simulink model "ModeAdjust"  (R2018b)
settings: Solver=FixedStepDiscrete  StartTime=0.0  StopTime=inf  FixedStep=0.01  RelTol=1e-3
undefined symbols (not defined in the file or in its folder): IfKeSMSbSeatMovBkRclnEnable_Val, IfKeSMSbSeatMovFrwdBkwdEnable_Val, IfKeSMSbSeatMovFtrstEnable_Val, IfKeSMSbSeatMovHdrstFrwdBkwdEnable_Val, IfKeSMSbSeatMovHdUpwdDnwdEnable_Val, IfKeSMSbSeatMovLgrstEnable_Val, IfKeSMSbSeatMovLtwdRtwdEnable_Val, IfVeSMSeStNumConfig, KeSMSbArmscreenMovEnable_Val, KeSMSbSeatMovLgrstExpdEnable_Val, KeSMSuFirstRwStBackPosDelta_Val, KeSMSuFirstRwStBackPosTolr_Val, KeSMSuFirstRwStCushFrntPosDelta_Val, KeSMSuFirstRwStCushFrntPosTolr_Val, KeSMSuFirstRwStCushRePosDelta_Val, KeSMSuFirstRwStCushRePosTolr_Val, KeSMSuFirstRwStFootrestPosDelta_Val, KeSMSuFirstRwStFootrestPosTolr_Val, KeSMSuFirstRwStFwdBkwdPosDelta_Val, KeSMSuFirstRwStFwdBkwdPosTolr_Val, KeSMSuMdMotFinshdTm_Val, KeSMSuMdRetryTm1_Val, KeSMSuModeReqDurgTm_Val, KeSMSuSecRwStArmTochPosDelta_Val, KeSMSuSecRwStArmTochPosTolr_Val, KeSMSuSecRwStBackPosDelta_Val, KeSMSuSecRwStBackPosTolr_Val, KeSMSuSecRwStFtrstUpwdDnwdPosDelta_Val, KeSMSuSecRwStFtrstUpwdDnwdPosTolr_Val, KeSMSuSecRwStFwdBkwdPosDelta_Val, KeSMSuSecRwStFwdBkwdPosTolr_Val, KeSMSuSecRwStHeadrestFwdBkwdPosDelta_Val, KeSMSuSecRwStHeadrestFwdBkwdPosTolr_Val, KeSMSuSecRwStHeadrestUpwdDwnwdPosDelta_Val, KeSMSuSecRwStHeadrestUpwdDwnwdPosTolr_Val, KeSMSuSecRwStLegrestInOutPosDelta_Val, KeSMSuSecRwStLegrestInOutPosTolr_Val, KeSMSuSecRwStLegrestUpwdDwnwdPosDelta_Val, KeSMSuSecRwStLegrestUpwdDwnwdPosTolr_Val, KeSMSuSecRwStLwdRwdPosDelta_Val, KeSMSuSecRwStLwdRwdPosTolr_Val, KeSMSuSecRwStVIPFtrstRefAngle_Val, KeSMSuThirdRwStFwdBkwdPosDelta_Val, KeSMSuThirdRwStFwdBkwdPosTolr_Val, KeSMSuThrdRwCushFoldPosDelta_Val, KeSMSuThrdRwCushFoldPosTolr_Val, KeSMSuThrdRwStBackPosDelta_Val, KeSMSuThrdRwStBackPosTolr_Val, KeSMSw4SLegrstCloseMdSecRwLtStFtrstUpwdDnwdPos_Val, KeSMSw4SLegrstCloseMdSecRwLtStFtrstUpwdDnwdPosMax_Val, KeSMSw4SLegrstCloseMdSecRwLtStFtrstUpwdDnwdPosMin_Val, KeSMSw4SLegrstCloseMdSecRwLtStLgrstOtwdInwdPos_Val, KeSMSw4SLegrstCloseMdSecRwLtStLgrstOtwdInwdPosMax_Val, KeSMSw4SLegrstCloseMdSecRwLtStLgrstOtwdInwdPosMin_Val, KeSMSw4SLegrstCloseMdSecRwLtStLgrstUpwdDnwdPos_Val, KeSMSw4SLegrstCloseMdSecRwLtStLgrstUpwdDnwdPosMax_Val, KeSMSw4SLegrstCloseMdSecRwLtStLgrstUpwdDnwdPosMin_Val, KeSMSw4SLegrstCloseMdSecRwRtStFtrstUpwdDnwdPos_Val, KeSMSw4SLegrstCloseMdSecRwRtStFtrstUpwdDnwdPosMax_Val, KeSMSw4SLegrstCloseMdSecRwRtStFtrstUpwdDnwdPosMin_Val ... (+1138)
libraries: Lib x401
(part 28 of 35)

== system ModeAdjust/ModeAdjustRunnable_sys/ModeAdjust/ArrivedAtTargetPosChk/Lug/R3Lt ==
  ThdRwLtStPoss : Inport
  ModeStCalib_3L : Inport  Port=2
  is6s : Inport  Port=3
  StConfig : Inport  Port=4
  IfVeSMSbThdRwLtStFrwdCmdSrv_Val_read : Inport  Port=5
  ThdRwLtStPossV : Inport  Port=6
  PosDeltaCalib : Inport  Port=7
  Bus Selector : BusSelector  OutputSignals=IfVeSMSuThdRwLtStBkReclnUpwdDnwdPos_Val_read,IfVeSMSuThdRwLtStCshnFldUpwdDnwdPos_Val_read,IfVeSMSuThdRwLtStFrwdBkwdPos_Val_read
  Bus Selector1 : BusSelector  OutputSignals=IfVeSMSuThdRwLtStBkReclnUpwdDnwdPosV_Val_read,IfVeSMSuThdRwLtStCshnFldUpwdDnwdPosV_Val_read,IfVeSMSuThdRwLtStFrwdBkwdPosV_Val_read
  Bus Selector2 : BusSelector  OutputSignals=BkReclnUpwdDnwdPos,BkReclnUpwdDnwdPosMax,BkReclnUpwdDnwdPosMin,CshnFldUpwdDnwdPos,CshnFldUpwdDnwdPosMax,CshnFldUpwdDnwdPosMin,FrwdBkwdPos,FrwdBkwdPosMax,FrwdBkwdPosMin
  Bus Selector3 : BusSelector  OutputSignals=LugThdRwLtSt
  Bus Selector4 : BusSelector  OutputSignals=BkReclnUpwdDnwdMovConfig,CshnFldUpwdDnwdMovConfig,FrwdBkwdMovConfig
  Bus Selector5 : BusSelector  OutputSignals=KeSMSuThirdRwStFwdBkwdPosDelta_Val,KeSMSuThrdRwCushFoldPosDelta_Val,KeSMSuThrdRwStBackPosDelta_Val
  CheckAtPos : Lib/CheckAtPos  SystemSampleTime=-1
  CheckAtPos1 : Lib/CheckAtPos  SystemSampleTime=-1
  CheckAtPos2 : Lib/CheckAtPos  SystemSampleTime=-1
  Constant{,1..4} (5 alike) : Constant  Value=0  OutDataTypeStr=boolean
  IsArrivedTarZone : Lib/CommonUsed/IniPosjudg/Subsystem2  SystemSampleTime=-1
  IsArrivedTarZone2 : Lib/CommonUsed/IniPosjudg/Subsystem2  SystemSampleTime=-1
  Logical Operator1 : Logic  Operator=NOT  AllPortsSameDT=off  OutDataTypeStr=boolean
  Logical Operator3 : Logic  Inputs=3  AllPortsSameDT=off  OutDataTypeStr=boolean
  R3Lt_ArrivedTarPos : Outport
  wires:
  Logical Operator3/1 -> R3Lt_ArrivedTarPos/1
  Bus Selector/1 -> [ThdRwLtStBkReclnUpwdDnwdPos]  "<IfVeSMSuThdRwLtStBkReclnUpwdDnwdPos_Val_read>"
  Bus Selector/3 -> [ThdRwLtStFrwdBkwdPos]  "<IfVeSMSuThdRwLtStFrwdBkwdPos_Val_read>"
  ThdRwLtStPoss/1 -> Bus Selector/1
  Bus Selector/2 -> [ThdRwLtStCshnFldUpwdDnwdPos]  "<IfVeSMSuThdRwLtStCshnFldUpwdDnwdPos_Val_read>"
  IsArrivedTarZone2/1 -> [Step3ArrivedTarPos]
  [ThdRwLtStCshnFldUpwdDnwdPos] -> IsArrivedTarZone2/1
  [K_CshnFldUpwdDnwdPosMin] -> IsArrivedTarZone2/2
  IsArrivedTarZone/1 -> [Step1ArrivedTarPos]
  [ThdRwLtStBkReclnUpwdDnwdPos] -> IsArrivedTarZone/1
  [K_BkReclnUpwdDnwdPosMin] -> IsArrivedTarZone/2
  [KeSMSuThrdRwStBackPosDelta_Val] -> IsArrivedTarZone/3
  [KeSMSuThrdRwCushFoldPosDelta_Val] -> IsArrivedTarZone2/3
  [K_BkReclnUpwdDnwdPosMax] -> IsArrivedTarZone/4
  [K_CshnFldUpwdDnwdPosMax] -> IsArrivedTarZone2/4
  Bus Selector2/6 -> [K_CshnFldUpwdDnwdPosMin]  "<CshnFldUpwdDnwdPosMin>"
  Bus Selector2/4 -> [K_CshnFldUpwdDnwdPos]  "<CshnFldUpwdDnwdPos>"
  Bus Selector2/7 -> [K_FrwdBkwdPos]  "<FrwdBkwdPos>"
  Bus Selector2/5 -> [K_CshnFldUpwdDnwdPosMax]  "<CshnFldUpwdDnwdPosMax>"
  ModeStCalib_3L/1 -> Bus Selector3/1
  Bus Selector2/3 -> [K_BkReclnUpwdDnwdPosMin]  "<BkReclnUpwdDnwdPosMin>"
  Bus Selector3/1 -> Bus Selector2/1  "<LugThdRwLtSt>"
  Bus Selector2/9 -> [K_FrwdBkwdPosMin]  "<FrwdBkwdPosMin>"
  Bus Selector2/2 -> [K_BkReclnUpwdDnwdPosMax]  "<BkReclnUpwdDnwdPosMax>"
  Bus Selector2/1 -> [K_BkReclnUpwdDnwdPos]  "<BkReclnUpwdDnwdPos>"
  Bus Selector2/8 -> [K_FrwdBkwdPosMax]  "<FrwdBkwdPosMax>"
  is6s/1 -> [is6s]
  Bus Selector4/1 -> [BkReclnUpwdDnwdMovConfig]  "<BkReclnUpwdDnwdMovConfig>"
  StConfig/1 -> Bus Selector4/1
  Bus Selector4/2 -> [CshnFldUpwdDnwdMovConfig]  "<CshnFldUpwdDnwdMovConfig>"
  Bus Selector4/3 -> [FrwdBkwdMovConfig]  "<FrwdBkwdMovConfig>"
  IfVeSMSbThdRwLtStFrwdCmdSrv_Val_read/1 -> Logical Operator1/1
  ThdRwLtStPossV/1 -> Bus Selector1/1
  Bus Selector1/3 -> [ThdRwLtStFrwdBkwdPosV]  "<IfVeSMSuThdRwLtStFrwdBkwdPosV_Val_read>"
  Bus Selector1/2 -> [ThdRwLtStCshnFldUpwdDnwdPosV]  "<IfVeSMSuThdRwLtStCshnFldUpwdDnwdPosV_Val_read>"
  Bus Selector1/1 -> [ThdRwLtStBkReclnUpwdDnwdPosV]  "<IfVeSMSuThdRwLtStBkReclnUpwdDnwdPosV_Val_read>"
  [BkReclnUpwdDnwdMovConfig] -> CheckAtPos/1
  [Step1ArrivedTarPos] -> CheckAtPos/3
  [FrwdBkwdMovConfig] -> CheckAtPos1/1
  Logical Operator1/1 -> CheckAtPos1/3
  [CshnFldUpwdDnwdMovConfig] -> CheckAtPos2/1
  [is6s] -> CheckAtPos2/5
  [Step3ArrivedTarPos] -> CheckAtPos2/3
  CheckAtPos1/1 -> Logical Operator3/2
  CheckAtPos2/1 -> Logical Operator3/3
  CheckAtPos/1 -> Logical Operator3/1
  [ThdRwLtStBkReclnUpwdDnwdPosV] -> CheckAtPos/2
  [ThdRwLtStCshnFldUpwdDnwdPosV] -> CheckAtPos2/2
  [ThdRwLtStFrwdBkwdPosV] -> CheckAtPos1/2
  Constant/1 -> CheckAtPos/4
  Constant1/1 -> CheckAtPos/5
  Constant2/1 -> CheckAtPos1/4
  Constant3/1 -> CheckAtPos1/5
  Constant4/1 -> CheckAtPos2/4
  Bus Selector5/1 -> [KeSMSuThirdRwStFwdBkwdPosDelta_Val]  "<KeSMSuThirdRwStFwdBkwdPosDelta_Val>"
  Bus Selector5/2 -> [KeSMSuThrdRwCushFoldPosDelta_Val]  "<KeSMSuThrdRwCushFoldPosDelta_Val>"
  Bus Selector5/3 -> [KeSMSuThrdRwStBackPosDelta_Val]  "<KeSMSuThrdRwStBackPosDelta_Val>"
  PosDeltaCalib/1 -> Bus Selector5/1

== system ModeAdjust/ModeAdjustRunnable_sys/ModeAdjust/ArrivedAtTargetPosChk/Lug/R3Rt ==
  ThdRwRtStPoss : Inport
  ModeStCalib_3R : Inport  Port=2
  is6s : Inport  Port=3
  StConfig : Inport  Port=4
  IfVeSMSbThdRwRtStFrwdCmdSrv_Val_read : Inport  Port=5
  ThdRwRtStPossV : Inport  Port=6
  PosDeltaCalib : Inport  Port=7
  Bus Selector : BusSelector  OutputSignals=IfVeSMSuThdRwRtStBkReclnUpwdDnwdPos_Val_read,IfVeSMSuThdRwRtStCshnFldUpwdDnwdPos_Val_read,IfVeSMSuThdRwRtStFrwdBkwdPos_Val_read
  Bus Selector1 : BusSelector  OutputSignals=IfVeSMSuThdRwRtStBkReclnUpwdDnwdPosV_Val_read,IfVeSMSuThdRwRtStCshnFldUpwdDnwdPosV_Val_read,IfVeSMSuThdRwRtStFrwdBkwdPosV_Val_read
  Bus Selector2 : BusSelector  OutputSignals=BkReclnUpwdDnwdPos,BkReclnUpwdDnwdPosMax,BkReclnUpwdDnwdPosMin,CshnFldUpwdDnwdPos,CshnFldUpwdDnwdPosMax,CshnFldUpwdDnwdPosMin,FrwdBkwdPos,FrwdBkwdPosMax,FrwdBkwdPosMin
  Bus Selector3 : BusSelector  OutputSignals=LugThdRwRtSt
  Bus Selector4 : BusSelector  OutputSignals=BkReclnUpwdDnwdMovConfig,CshnFldUpwdDnwdMovConfig,FrwdBkwdMovConfig
  Bus Selector5 : BusSelector  OutputSignals=KeSMSuThirdRwStFwdBkwdPosDelta_Val,KeSMSuThrdRwCushFoldPosDelta_Val,KeSMSuThrdRwStBackPosDelta_Val
  CheckAtPos : Lib/CheckAtPos  SystemSampleTime=-1
  CheckAtPos1 : Lib/CheckAtPos  SystemSampleTime=-1
  CheckAtPos2 : Lib/CheckAtPos  SystemSampleTime=-1
  Constant{,1..4} (5 alike) : Constant  Value=0  OutDataTypeStr=boolean
  IsArrivedTarZone : Lib/CommonUsed/IniPosjudg/Subsystem2  SystemSampleTime=-1
  IsArrivedTarZone2 : Lib/CommonUsed/IniPosjudg/Subsystem2  SystemSampleTime=-1
  Logical Operator1 : Logic  Operator=NOT  AllPortsSameDT=off  OutDataTypeStr=boolean
  Logical Operator3 : Logic  Inputs=3  AllPortsSameDT=off  OutDataTypeStr=boolean
  R3Rt_ArrivedTarPos : Outport
  wires:
  Logical Operator3/1 -> R3Rt_ArrivedTarPos/1
  Bus Selector/1 -> [ThdRwRtStBkReclnUpwdDnwdPos]  "<IfVeSMSuThdRwRtStBkReclnUpwdDnwdPos_Val_read>"
  Bus Selector/2 -> [ThdRwRtStCshnFldUpwdDnwdPos]  "<IfVeSMSuThdRwRtStCshnFldUpwdDnwdPos_Val_read>"
  ThdRwRtStPoss/1 -> Bus Selector/1
  Bus Selector/3 -> [ThdRwRtStFrwdBkwdPos]  "<IfVeSMSuThdRwRtStFrwdBkwdPos_Val_read>"
  [ThdRwRtStBkReclnUpwdDnwdPos] -> IsArrivedTarZone/1
  IsArrivedTarZone/1 -> [Step1ArrivedTarPos]
  [K_CshnFldUpwdDnwdPosMin] -> IsArrivedTarZone2/2
  [ThdRwRtStCshnFldUpwdDnwdPos] -> IsArrivedTarZone2/1
  IsArrivedTarZone2/1 -> [Step3ArrivedTarPos]
  [K_BkReclnUpwdDnwdPosMin] -> IsArrivedTarZone/2
  [KeSMSuThrdRwStBackPosDelta_Val] -> IsArrivedTarZone/3
  [KeSMSuThrdRwCushFoldPosDelta_Val] -> IsArrivedTarZone2/3
  [K_BkReclnUpwdDnwdPosMax] -> IsArrivedTarZone/4
  [K_CshnFldUpwdDnwdPosMax] -> IsArrivedTarZone2/4
  Bus Selector2/6 -> [K_CshnFldUpwdDnwdPosMin]  "<CshnFldUpwdDnwdPosMin>"
  Bus Selector2/4 -> [K_CshnFldUpwdDnwdPos]  "<CshnFldUpwdDnwdPos>"
  Bus Selector2/7 -> [K_FrwdBkwdPos]  "<FrwdBkwdPos>"
  Bus Selector2/5 -> [K_CshnFldUpwdDnwdPosMax]  "<CshnFldUpwdDnwdPosMax>"
  ModeStCalib_3R/1 -> Bus Selector3/1
  Bus Selector2/3 -> [K_BkReclnUpwdDnwdPosMin]  "<BkReclnUpwdDnwdPosMin>"
  Bus Selector3/1 -> Bus Selector2/1  "<LugThdRwRtSt>"
  Bus Selector2/9 -> [K_FrwdBkwdPosMin]  "<FrwdBkwdPosMin>"
  Bus Selector2/2 -> [K_BkReclnUpwdDnwdPosMax]  "<BkReclnUpwdDnwdPosMax>"
  Bus Selector2/1 -> [K_BkReclnUpwdDnwdPos]  "<BkReclnUpwdDnwdPos>"
  Bus Selector2/8 -> [K_FrwdBkwdPosMax]  "<FrwdBkwdPosMax>"
  is6s/1 -> [is6s]
  Bus Selector4/1 -> [BkReclnUpwdDnwdMovConfig]  "<BkReclnUpwdDnwdMovConfig>"
  StConfig/1 -> Bus Selector4/1
  Bus Selector4/2 -> [CshnFldUpwdDnwdMovConfig]  "<CshnFldUpwdDnwdMovConfig>"
  Bus Selector4/3 -> [FrwdBkwdMovConfig]  "<FrwdBkwdMovConfig>"
  IfVeSMSbThdRwRtStFrwdCmdSrv_Val_read/1 -> Logical Operator1/1
  ThdRwRtStPossV/1 -> Bus Selector1/1
  Bus Selector1/1 -> [ThdRwRtStBkReclnUpwdDnwdPosV]  "<IfVeSMSuThdRwRtStBkReclnUpwdDnwdPosV_Val_read>"
  Bus Selector1/3 -> [ThdRwRtStFrwdBkwdPosV]  "<IfVeSMSuThdRwRtStFrwdBkwdPosV_Val_read>"
  Bus Selector1/2 -> [ThdRwRtStCshnFldUpwdDnwdPosV]  "<IfVeSMSuThdRwRtStCshnFldUpwdDnwdPosV_Val_read>"
  CheckAtPos1/1 -> Logical Operator3/2
  CheckAtPos2/1 -> Logical Operator3/3
  CheckAtPos/1 -> Logical Operator3/1
  [BkReclnUpwdDnwdMovConfig] -> CheckAtPos/1
  [Step1ArrivedTarPos] -> CheckAtPos/3
  Logical Operator1/1 -> CheckAtPos1/3
  [FrwdBkwdMovConfig] -> CheckAtPos1/1
  [CshnFldUpwdDnwdMovConfig] -> CheckAtPos2/1
  [is6s] -> CheckAtPos2/5
  [Step3ArrivedTarPos] -> CheckAtPos2/3
  [ThdRwRtStBkReclnUpwdDnwdPosV] -> CheckAtPos/2
  [ThdRwRtStCshnFldUpwdDnwdPosV] -> CheckAtPos2/2
  [ThdRwRtStFrwdBkwdPosV] -> CheckAtPos1/2
  Constant/1 -> CheckAtPos/4
  Constant1/1 -> CheckAtPos/5
  Constant2/1 -> CheckAtPos1/4
  Constant3/1 -> CheckAtPos1/5
  Constant4/1 -> CheckAtPos2/4
  Bus Selector5/1 -> [KeSMSuThirdRwStFwdBkwdPosDelta_Val]  "<KeSMSuThirdRwStFwdBkwdPosDelta_Val>"
  Bus Selector5/2 -> [KeSMSuThrdRwCushFoldPosDelta_Val]  "<KeSMSuThrdRwCushFoldPosDelta_Val>"
  Bus Selector5/3 -> [KeSMSuThrdRwStBackPosDelta_Val]  "<KeSMSuThrdRwStBackPosDelta_Val>"
  PosDeltaCalib/1 -> Bus Selector5/1

== system ModeAdjust/ModeAdjustRunnable_sys/ModeAdjust/ArrivedAtTargetPosChk/Lug/Subsystem1 ==
  Left_inport : Inport
  Right_inport : Inport  Port=2
  Md_L_MvDoneOK : Outport
  Md_R_MvDoneOK : Outport  Port=2
  wires:
  Left_inport/1 -> Md_L_MvDoneOK/1
  Right_inport/1 -> Md_R_MvDoneOK/1

== system ModeAdjust/ModeAdjustRunnable_sys/ModeAdjust/ArrivedAtTargetPosChk/Ly/R2Lt ==
  SecRwLtStsPoss : Inport
  ModeStCalib_2L : Inport  Port=2
  StConfig : Inport  Port=3
  SecRwLtStsPoss4s : Inport  Port=4
  StConfig4s : Inport  Port=5
  SecRwLtStPossV : Inport  Port=6
  SecRwLtStPossV4s : Inport  Port=7
  Lt4sHightIndex : Inport  Port=8
  PosDeltaCalib : Inport  Port=9
  Bus Creator{,1..6} (7 alike) : BusCreator  Inputs=9
  Bus Selector : BusSelector  OutputSignals=IfVeSMSuSecRwLtStBkReclnUpwdDnwdPos_Val_read,IfVeSMSuSecRwLtStFrwdBkwdPos_Val_read,IfVeSMSuSecRwLtStHPassStUpwdDnwdPos_Val_read,IfVeSMSuSecRwLtStLgrstUpwdDnwdPos_Val_read,IfVeSMSuSecRwLtStLtwdRtwdPos_Val_read,IfVeSMSuSecRwLtStArmScrnPos_Val_read
  Bus Selector1 : BusSelector  OutputSignals=IfVeSMSuSecRwLtStLgrstOtwdInwdPos_Val_read,IfVeSMSuRrLtStFtUpwdDnwdPos_Val_read,IfVeSMSuSecRwLtStHdrstFrwdBkwdPos_Val_read
  Bus Selector2 : BusSelector  OutputSignals=BkReclnUpwdDnwdPosMax,BkReclnUpwdDnwdPosMin,LgrstUpwdPosMax,LgrstUpwdPosMin,FtrstUpwdDnwdPosMax,FtrstUpwdDnwdPosMin
  Bus Selector3 : BusSelector  OutputSignals=LyLSecRwLtSt
  Bus Selector4 : BusSelector  OutputSignals=BkReclnUpwdDnwdMovConfig,ArmTouchMovConfig,FrwdBkwdMovConfig,LgrstUpwdMovConfig,LtwdRtwdMovConfig
  Bus Selector5 : BusSelector  OutputSignals=LgrstExpdMovConfig,FtrstMovConfig,HdrstUpwdDnwdMovConfig,HdrstFrwdBkwdMovConfig
  Bus Selector6 : BusSelector  OutputSignals=IfVeSMSuSecRwLtStBkReclnUpwdDnwdPosV_Val_read,IfVeSMSuSecRwLtStFrwdBkwdPosV_Val_read,IfVeSMSuSecRwLtStHPassStUpwdDnwdPosV_Val_read,IfVeSMSuSecRwLtStLgrstUpwdDnwdPosV_Val_read,IfVeSMSuSecRwLtStLtwdRtwdPosV_Val_read,IfVeSMSuSecRwLtStArmScrnPosV_Val_read
  Bus Selector7 : BusSelector  OutputSignals=IfVeSMSuSecRwLtStLgrstOtwdInwdPosV_Val_read,IfVeSMSuRrLtStFtUpwdDnwdPosV_Val_read,IfVeSMSuSecRwLtStHdrstFrwdBkwdPosV_Val_read
  Bus Selector8 : BusSelector  OutputSignals=HdrstUpwdDnwdPosMax,HdrstUpwdDnwdPosMin,HdrstFrwdBkwdnwdPosMax,HdrstFrwdBkwdnwdPosMin,LgrstOtwdInwdPosMax,LgrstOtwdInwdPosMin
  Bus Selector9 : BusSelector  OutputSignals=KeSMSuSecRwStHeadrestFwdBkwdPosDelta_Val,KeSMSuSecRwStHeadrestUpwdDwnwdPosDelta_Val,KeSMSuSecRwStLegrestInOutPosDelta_Val,KeSMSuSecRwStFtrstUpwdDnwdPosDelta_Val,KeSMSuSecRwStBackPosDelta_Val,KeSMSuSecRwStLegrestUpwdDwnwdPosDelta_Val
  CheckAtPos{,1..5} (6 alike) : Lib/CheckAtPos  SystemSampleTime=-1
  Constant{1..12} (12 alike) : Constant  Value=0  OutDataTypeStr=boolean
  IsArrivedTarZone{,1..5} (6 alike) : Lib/CommonUsed/IniPosjudg/Subsystem2  SystemSampleTime=-1
  Logical Operator9 : Logic  Inputs=6  AllPortsSameDT=off  OutDataTypeStr=boolean
  Multiport Switch : MultiPortSwitch  DataPortOrder=Zero-based contiguous  Inputs=7  DiagnosticForDefault=None  zeroidx=on
  PA_KeSMSw4sLyingMDSecRwLtStHdrstFrwdBkwdnwdPosMax_160_Val : Constant  Value=KeSMSw4sLyingMDSecRwLtStHdrstFrwdBkwdnwdPosMax_160_Val
  PA_KeSMSw4sLyingMDSecRwLtStHdrstFrwdBkwdnwdPosMax_165_Val : Constant  Value=KeSMSw4sLyingMDSecRwLtStHdrstFrwdBkwdnwdPosMax_165_Val
  PA_KeSMSw4sLyingMDSecRwLtStHdrstFrwdBkwdnwdPosMax_170_Val : Constant  Value=KeSMSw4sLyingMDSecRwLtStHdrstFrwdBkwdnwdPosMax_170_Val
  PA_KeSMSw4sLyingMDSecRwLtStHdrstFrwdBkwdnwdPosMax_175_Val : Constant  Value=KeSMSw4sLyingMDSecRwLtStHdrstFrwdBkwdnwdPosMax_175_Val
  PA_KeSMSw4sLyingMDSecRwLtStHdrstFrwdBkwdnwdPosMax_180_Val : Constant  Value=KeSMSw4sLyingMDSecRwLtStHdrstFrwdBkwdnwdPosMax_180_Val
  PA_KeSMSw4sLyingMDSecRwLtStHdrstFrwdBkwdnwdPosMax_Below160_Val : Constant  Value=KeSMSw4sLyingMDSecRwLtStHdrstFrwdBkwdnwdPosMax_Below160_Val
  PA_KeSMSw4sLyingMDSecRwLtStHdrstFrwdBkwdnwdPosMax_Over180_Val : Constant  Value=KeSMSw4sLyingMDSecRwLtStHdrstFrwdBkwdnwdPosMax_Over180_Val
  PA_KeSMSw4sLyingMDSecRwLtStHdrstFrwdBkwdnwdPosMin_160_Val : Constant  Value=KeSMSw4sLyingMDSecRwLtStHdrstFrwdBkwdnwdPosMin_160_Val
  PA_KeSMSw4sLyingMDSecRwLtStHdrstFrwdBkwdnwdPosMin_165_Val : Constant  Value=KeSMSw4sLyingMDSecRwLtStHdrstFrwdBkwdnwdPosMin_165_Val
  PA_KeSMSw4sLyingMDSecRwLtStHdrstFrwdBkwdnwdPosMin_170_Val : Constant  Value=KeSMSw4sLyingMDSecRwLtStHdrstFrwdBkwdnwdPosMin_170_Val
  PA_KeSMSw4sLyingMDSecRwLtStHdrstFrwdBkwdnwdPosMin_175_Val : Constant  Value=KeSMSw4sLyingMDSecRwLtStHdrstFrwdBkwdnwdPosMin_175_Val
  PA_KeSMSw4sLyingMDSecRwLtStHdrstFrwdBkwdnwdPosMin_180_Val : Constant  Value=KeSMSw4sLyingMDSecRwLtStHdrstFrwdBkwdnwdPosMin_180_Val
  PA_KeSMSw4sLyingMDSecRwLtStHdrstFrwdBkwdnwdPosMin_Below160_Val : Constant  Value=KeSMSw4sLyingMDSecRwLtStHdrstFrwdBkwdnwdPosMin_Below160_Val
  PA_KeSMSw4sLyingMDSecRwLtStHdrstFrwdBkwdnwdPosMin_Over180_Val : Constant  Value=KeSMSw4sLyingMDSecRwLtStHdrstFrwdBkwdnwdPosMin_Over180_Val
  PA_KeSMSw4sLyingMDSecRwLtStHdrstFrwdBkwdnwdPos_160_Val : Constant  Value=KeSMSw4sLyingMDSecRwLtStHdrstFrwdBkwdnwdPos_160_Val
  PA_KeSMSw4sLyingMDSecRwLtStHdrstFrwdBkwdnwdPos_165_Val : Constant  Value=KeSMSw4sLyingMDSecRwLtStHdrstFrwdBkwdnwdPos_165_Val
  PA_KeSMSw4sLyingMDSecRwLtStHdrstFrwdBkwdnwdPos_170_Val : Constant  Value=KeSMSw4sLyingMDSecRwLtStHdrstFrwdBkwdnwdPos_170_Val
  PA_KeSMSw4sLyingMDSecRwLtStHdrstFrwdBkwdnwdPos_175_Val : Constant  Value=KeSMSw4sLyingMDSecRwLtStHdrstFrwdBkwdnwdPos_175_Val
  PA_KeSMSw4sLyingMDSecRwLtStHdrstFrwdBkwdnwdPos_180_Val : Constant  Value=KeSMSw4sLyingMDSecRwLtStHdrstFrwdBkwdnwdPos_180_Val
  PA_KeSMSw4sLyingMDSecRwLtStHdrstFrwdBkwdnwdPos_Below160_Val : Constant  Value=KeSMSw4sLyingMDSecRwLtStHdrstFrwdBkwdnwdPos_Below160_Val
  PA_KeSMSw4sLyingMDSecRwLtStHdrstFrwdBkwdnwdPos_Over180_Val : Constant  Value=KeSMSw4sLyingMDSecRwLtStHdrstFrwdBkwdnwdPos_Over180_Val
  PA_KeSMSw4sLyingMDSecRwLtStHdrstUpwdDnwdPosMax_160_Val : Constant  Value=KeSMSw4sLyingMDSecRwLtStHdrstUpwdDnwdPosMax_160_Val
  PA_KeSMSw4sLyingMDSecRwLtStHdrstUpwdDnwdPosMax_165_Val : Constant  Value=KeSMSw4sLyingMDSecRwLtStHdrstUpwdDnwdPosMax_165_Val
  PA_KeSMSw4sLyingMDSecRwLtStHdrstUpwdDnwdPosMax_170_Val : Constant  Value=KeSMSw4sLyingMDSecRwLtStHdrstUpwdDnwdPosMax_170_Val
  PA_KeSMSw4sLyingMDSecRwLtStHdrstUpwdDnwdPosMax_175_Val : Constant  Value=KeSMSw4sLyingMDSecRwLtStHdrstUpwdDnwdPosMax_175_Val
  PA_KeSMSw4sLyingMDSecRwLtStHdrstUpwdDnwdPosMax_180_Val : Constant  Value=KeSMSw4sLyingMDSecRwLtStHdrstUpwdDnwdPosMax_180_Val
  PA_KeSMSw4sLyingMDSecRwLtStHdrstUpwdDnwdPosMax_Below160_Val : Constant  Value=KeSMSw4sLyingMDSecRwLtStHdrstUpwdDnwdPosMax_Below160_Val
  PA_KeSMSw4sLyingMDSecRwLtStHdrstUpwdDnwdPosMax_Over180_Val : Constant  Value=KeSMSw4sLyingMDSecRwLtStHdrstUpwdDnwdPosMax_Over180_Val
  PA_KeSMSw4sLyingMDSecRwLtStHdrstUpwdDnwdPosMin_160_Val : Constant  Value=KeSMSw4sLyingMDSecRwLtStHdrstUpwdDnwdPosMin_160_Val
  PA_KeSMSw4sLyingMDSecRwLtStHdrstUpwdDnwdPosMin_165_Val : Constant  Value=KeSMSw4sLyingMDSecRwLtStHdrstUpwdDnwdPosMin_165_Val
  PA_KeSMSw4sLyingMDSecRwLtStHdrstUpwdDnwdPosMin_170_Val : Constant  Value=KeSMSw4sLyingMDSecRwLtStHdrstUpwdDnwdPosMin_170_Val
  PA_KeSMSw4sLyingMDSecRwLtStHdrstUpwdDnwdPosMin_175_Val : Constant  Value=KeSMSw4sLyingMDSecRwLtStHdrstUpwdDnwdPosMin_175_Val
  PA_KeSMSw4sLyingMDSecRwLtStHdrstUpwdDnwdPosMin_180_Val : Constant  Value=KeSMSw4sLyingMDSecRwLtStHdrstUpwdDnwdPosMin_180_Val
  PA_KeSMSw4sLyingMDSecRwLtStHdrstUpwdDnwdPosMin_Below160_Val : Constant  Value=KeSMSw4sLyingMDSecRwLtStHdrstUpwdDnwdPosMin_Below160_Val
  PA_KeSMSw4sLyingMDSecRwLtStHdrstUpwdDnwdPosMin_Over180_Val : Constant  Value=KeSMSw4sLyingMDSecRwLtStHdrstUpwdDnwdPosMin_Over180_Val
  PA_KeSMSw4sLyingMDSecRwLtStHdrstUpwdDnwdPos_160_Val : Constant  Value=KeSMSw4sLyingMDSecRwLtStHdrstUpwdDnwdPos_160_Val
  PA_KeSMSw4sLyingMDSecRwLtStHdrstUpwdDnwdPos_165_Val : Constant  Value=KeSMSw4sLyingMDSecRwLtStHdrstUpwdDnwdPos_165_Val
  PA_KeSMSw4sLyingMDSecRwLtStHdrstUpwdDnwdPos_170_Val : Constant  Value=KeSMSw4sLyingMDSecRwLtStHdrstUpwdDnwdPos_170_Val
  PA_KeSMSw4sLyingMDSecRwLtStHdrstUpwdDnwdPos_175_Val : Constant  Value=KeSMSw4sLyingMDSecRwLtStHdrstUpwdDnwdPos_175_Val
  PA_KeSMSw4sLyingMDSecRwLtStHdrstUpwdDnwdPos_180_Val : Constant  Value=KeSMSw4sLyingMDSecRwLtStHdrstUpwdDnwdPos_180_Val
  PA_KeSMSw4sLyingMDSecRwLtStHdrstUpwdDnwdPos_Below160_Val : Constant  Value=KeSMSw4sLyingMDSecRwLtStHdrstUpwdDnwdPos_Below160_Val
  PA_KeSMSw4sLyingMDSecRwLtStHdrstUpwdDnwdPos_Over180_Val : Constant  Value=KeSMSw4sLyingMDSecRwLtStHdrstUpwdDnwdPos_Over180_Val
  PA_KeSMSw4sLyingMDSecRwLtStLgrstOtwdInwdPosMax_160_Val : Constant  Value=KeSMSw4sLyingMDSecRwLtStLgrstOtwdInwdPosMax_160_Val
  PA_KeSMSw4sLyingMDSecRwLtStLgrstOtwdInwdPosMax_165_Val : Constant  Value=KeSMSw4sLyingMDSecRwLtStLgrstOtwdInwdPosMax_165_Val
  PA_KeSMSw4sLyingMDSecRwLtStLgrstOtwdInwdPosMax_170_Val : Constant  Value=KeSMSw4sLyingMDSecRwLtStLgrstOtwdInwdPosMax_170_Val
  PA_KeSMSw4sLyingMDSecRwLtStLgrstOtwdInwdPosMax_175_Val : Constant  Value=KeSMSw4sLyingMDSecRwLtStLgrstOtwdInwdPosMax_175_Val
  PA_KeSMSw4sLyingMDSecRwLtStLgrstOtwdInwdPosMax_180_Val : Constant  Value=KeSMSw4sLyingMDSecRwLtStLgrstOtwdInwdPosMax_180_Val
  PA_KeSMSw4sLyingMDSecRwLtStLgrstOtwdInwdPosMax_Below160_Val : Constant  Value=KeSMSw4sLyingMDSecRwLtStLgrstOtwdInwdPosMax_Below160_Val
  PA_KeSMSw4sLyingMDSecRwLtStLgrstOtwdInwdPosMax_Over180_Val : Constant  Value=KeSMSw4sLyingMDSecRwLtStLgrstOtwdInwdPosMax_Over180_Val
  PA_KeSMSw4sLyingMDSecRwLtStLgrstOtwdInwdPosMin_160_Val : Constant  Value=KeSMSw4sLyingMDSecRwLtStLgrstOtwdInwdPosMin_160_Val
  PA_KeSMSw4sLyingMDSecRwLtStLgrstOtwdInwdPosMin_165_Val : Constant  Value=KeSMSw4sLyingMDSecRwLtStLgrstOtwdInwdPosMin_165_Val
  PA_KeSMSw4sLyingMDSecRwLtStLgrstOtwdInwdPosMin_170_Val : Constant  Value=KeSMSw4sLyingMDSecRwLtStLgrstOtwdInwdPosMin_170_Val
  PA_KeSMSw4sLyingMDSecRwLtStLgrstOtwdInwdPosMin_175_Val : Constant  Value=KeSMSw4sLyingMDSecRwLtStLgrstOtwdInwdPosMin_175_Val
  PA_KeSMSw4sLyingMDSecRwLtStLgrstOtwdInwdPosMin_180_Val : Constant  Value=KeSMSw4sLyingMDSecRwLtStLgrstOtwdInwdPosMin_180_Val
  PA_KeSMSw4sLyingMDSecRwLtStLgrstOtwdInwdPosMin_Below160_Val : Constant  Value=KeSMSw4sLyingMDSecRwLtStLgrstOtwdInwdPosMin_Below160_Val
  PA_KeSMSw4sLyingMDSecRwLtStLgrstOtwdInwdPosMin_Over180_Val : Constant  Value=KeSMSw4sLyingMDSecRwLtStLgrstOtwdInwdPosMin_Over180_Val
  PA_KeSMSw4sLyingMDSecRwLtStLgrstOtwdInwdPos_160_Val : Constant  Value=KeSMSw4sLyingMDSecRwLtStLgrstOtwdInwdPos_160_Val
  PA_KeSMSw4sLyingMDSecRwLtStLgrstOtwdInwdPos_165_Val : Constant  Value=KeSMSw4sLyingMDSecRwLtStLgrstOtwdInwdPos_165_Val
  PA_KeSMSw4sLyingMDSecRwLtStLgrstOtwdInwdPos_170_Val : Constant  Value=KeSMSw4sLyingMDSecRwLtStLgrstOtwdInwdPos_170_Val
  PA_KeSMSw4sLyingMDSecRwLtStLgrstOtwdInwdPos_175_Val : Constant  Value=KeSMSw4sLyingMDSecRwLtStLgrstOtwdInwdPos_175_Val
  PA_KeSMSw4sLyingMDSecRwLtStLgrstOtwdInwdPos_180_Val : Constant  Value=KeSMSw4sLyingMDSecRwLtStLgrstOtwdInwdPos_180_Val
  PA_KeSMSw4sLyingMDSecRwLtStLgrstOtwdInwdPos_Below160_Val : Constant  Value=KeSMSw4sLyingMDSecRwLtStLgrstOtwdInwdPos_Below160_Val
  PA_KeSMSw4sLyingMDSecRwLtStLgrstOtwdInwdPos_Over180_Val : Constant  Value=KeSMSw4sLyingMDSecRwLtStLgrstOtwdInwdPos_Over180_Val
  R2Lt_ArrivedTarPos : Outport
  Calib_Ly4sLAdpt : Outport  Port=2
  wires:
  IsArrivedTarZone/1 -> [Step1_1_ArrivedTarPos]
  [SecRwLtStBkReclnUpwdDnwdPos] -> IsArrivedTarZone/1
  [K_BkReclnUpwdDnwdPosMin] -> IsArrivedTarZone/2
  Bus Selector/5 -> [SecRwLtStLtwdRtwdPos]  "<IfVeSMSuSecRwLtStLtwdRtwdPos_Val_read>"
  SecRwLtStsPoss/1 -> Bus Selector/1
  Bus Selector/3 -> [SecRwLtStHPassStUpwdDnwdPos]  "<IfVeSMSuSecRwLtStHPassStUpwdDnwdPos_Val_read>"
  Bus Selector/4 -> [SecRwLtStLgrstUpwdDnwdPos]  "<IfVeSMSuSecRwLtStLgrstUpwdDnwdPos_Val_read>"
  Bus Selector/2 -> [SecRwLtStFrwdBkwdPos]  "<IfVeSMSuSecRwLtStFrwdBkwdPos_Val_read>"
  Bus Selector/1 -> [SecRwLtStBkReclnUpwdDnwdPos]  "<IfVeSMSuSecRwLtStBkReclnUpwdDnwdPos_Val_read>"
  [K_LgrstUpwdPosMin] -> IsArrivedTarZone1/2
  [SecRwLtStLgrstUpwdDnwdPos] -> IsArrivedTarZone1/1
  IsArrivedTarZone1/1 -> [Step1_2_ArrivedTarPos]
  Logical Operator9/1 -> R2Lt_ArrivedTarPos/1
  IsArrivedTarZone2/1 -> [Step1_3_ArrivedTarPos]
  Bus Selector/6 -> [SecRwLtStArmScrnPos]  "<IfVeSMSuSecRwLtStArmScrnPos_Val_read>"
  [KeSMSuSecRwStBackPosDelta_Val] -> IsArrivedTarZone/3
  [K_BkReclnUpwdDnwdPosMax] -> IsArrivedTarZone/4
  [K_LgrstUpwdPosMax] -> IsArrivedTarZone1/4
  [KeSMSuSecRwStLegrestUpwdDwnwdPosDelta_Val] -> IsArrivedTarZone1/3
  Bus Selector2/1 -> [K_BkReclnUpwdDnwdPosMax]  "<BkReclnUpwdDnwdPosMax>"
  Bus Selector3/1 -> Bus Selector2/1  "<LyLSecRwLtSt>"
  Bus Selector2/2 -> [K_BkReclnUpwdDnwdPosMin]  "<BkReclnUpwdDnwdPosMin>"
  ModeStCalib_2L/1 -> Bus Selector3/1
  StConfig/1 -> Bus Selector4/1
  Bus Selector4/3 -> [FrwdBkwdMovConfig]  "<FrwdBkwdMovConfig>"
  Bus Selector4/5 -> [LtwdRtwdMovConfig]  "<LtwdRtwdMovConfig>"
  Bus Selector4/4 -> [LgrstUpwdMovConfig]  "<LgrstUpwdMovConfig>"
  Bus Selector4/2 -> [ArmTouchMovConfig]  "<ArmTouchMovConfig>"
  Bus Selector4/1 -> [BkReclnUpwdDnwdMovConfig]  "<BkReclnUpwdDnwdMovConfig>"
  [K_HdrstUpwdPosMax] -> IsArrivedTarZone2/4
  [K_HdrstUpwdPosMin] -> IsArrivedTarZone2/2
  [SecRwLtStHPassStUpwdDnwdPos] -> IsArrivedTarZone2/1
  [KeSMSuSecRwStHeadrestUpwdDwnwdPosDelta_Val] -> IsArrivedTarZone2/3
  [KeSMSuSecRwStFtrstUpwdDnwdPosDelta_Val] -> IsArrivedTarZone3/3
  SecRwLtStsPoss4s/1 -> Bus Selector1/1
  Bus Selector1/1 -> [SecRwLtStLgrstOtwdInwdPos]  "<IfVeSMSuSecRwLtStLgrstOtwdInwdPos_Val_read>"
  Bus Selector1/2 -> [IfVeSMSuRrLtStFtUpwdDnwdPos]  "<IfVeSMSuRrLtStFtUpwdDnwdPos_Val_read>"
  [IfVeSMSuRrLtStFtUpwdDnwdPos] -> IsArrivedTarZone3/1
  Bus Selector2/5 -> [K_FtrstUpwdDnwdPos_Max]  "<FtrstUpwdDnwdPosMax>"
  Bus Selector2/6 -> [K_FtrstUpwdDnwdPos_Min]  "<FtrstUpwdDnwdPosMin>"
  [K_FtrstUpwdDnwdPos_Min] -> IsArrivedTarZone3/2
  [K_FtrstUpwdDnwdPos_Max] -> IsArrivedTarZone3/4
  IsArrivedTarZone3/1 -> [Step1_4_ArrivedTarPos]
  [K_LgrstOtwdInwdPos_Min] -> IsArrivedTarZone4/2
  [K_LgrstOtwdInwdPos_Max] -> IsArrivedTarZone4/4
  [SecRwLtStLgrstOtwdInwdPos] -> IsArrivedTarZone4/1
  [KeSMSuSecRwStLegrestInOutPosDelta_Val] -> IsArrivedTarZone4/3
  IsArrivedTarZone4/1 -> [Step1_5_ArrivedTarPos]
  StConfig4s/1 -> Bus Selector5/1
  Bus Selector5/3 -> [HdrstMovConfig]  "<HdrstUpwdDnwdMovConfig>"
  Bus Selector5/1 -> [LgrstExpdMovConfig]  "<LgrstExpdMovConfig>"
  Bus Selector5/2 -> [FtrstMovConfig]  "<FtrstMovConfig>"
  Bus Selector6/6 -> [IfVeSMSuSecRwLtStArmScrnPosV]  "<IfVeSMSuSecRwLtStArmScrnPosV_Val_read>"
  Bus Selector6/3 -> [SecRwLtStHPassStUpwdDnwdPosV]  "<IfVeSMSuSecRwLtStHPassStUpwdDnwdPosV_Val_read>"
  Bus Selector6/2 -> [SecRwLtStFrwdBkwdPosV]  "<IfVeSMSuSecRwLtStFrwdBkwdPosV_Val_read>"
  Bus Selector6/4 -> [SecRwLtStLgrstUpwdDnwdPosV]  "<IfVeSMSuSecRwLtStLgrstUpwdDnwdPosV_Val_read>"
  Bus Selector6/5 -> [SecRwLtStLtwdRtwdPosV]  "<IfVeSMSuSecRwLtStLtwdRtwdPosV_Val_read>"
  SecRwLtStPossV/1 -> Bus Selector6/1
  Bus Selector6/1 -> [SecRwLtStBkReclnUpwdDnwdPosV]  "<IfVeSMSuSecRwLtStBkReclnUpwdDnwdPosV_Val_read>"
  CheckAtPos3/1 -> Logical Operator9/4  "LyL_Step1_4_ArrivedTarPos"
  CheckAtPos/1 -> Logical Operator9/3  "LyL_Step1_3_ArrivedTarPos"
  CheckAtPos4/1 -> Logical Operator9/5  "LyL_Step1_5_ArrivedTarPos"
  CheckAtPos1/1 -> Logical Operator9/2  "LyL_Step1_2_ArrivedTarPos"
  CheckAtPos2/1 -> Logical Operator9/1  "LyL_Step1_1_ArrivedTarPos"
  [BkReclnUpwdDnwdMovConfig] -> CheckAtPos2/1
  [Step1_1_ArrivedTarPos] -> CheckAtPos2/3
  [LgrstUpwdMovConfig] -> CheckAtPos1/1
  [Step1_2_ArrivedTarPos] -> CheckAtPos1/3
  [HdrstMovConfig] -> CheckAtPos/1
  [Step1_3_ArrivedTarPos] -> CheckAtPos/3
  [FtrstMovConfig] -> CheckAtPos3/1
  [Step1_4_ArrivedTarPos] -> CheckAtPos3/3
  [LgrstExpdMovConfig] -> CheckAtPos4/1
  [Step1_5_ArrivedTarPos] -> CheckAtPos4/3
  [SecRwLtStLgrstUpwdDnwdPosV] -> CheckAtPos1/2
  SecRwLtStPossV4s/1 -> Bus Selector7/1
  Bus Selector7/2 -> [RrLtStFtUpwdDnwdPosV]  "<IfVeSMSuRrLtStFtUpwdDnwdPosV_Val_read>"
  Bus Selector7/1 -> [SecRwLtStLgrstOtwdInwdPosV]  "<IfVeSMSuSecRwLtStLgrstOtwdInwdPosV_Val_read>"
  [SecRwLtStHPassStUpwdDnwdPosV] -> CheckAtPos/2
  [RrLtStFtUpwdDnwdPosV] -> CheckAtPos3/2
  [SecRwLtStLgrstOtwdInwdPosV] -> CheckAtPos4/2
  Constant3/1 -> CheckAtPos2/5
  Constant2/1 -> CheckAtPos2/4
  Constant4/1 -> CheckAtPos1/5
  Constant1/1 -> CheckAtPos1/4
  Constant6/1 -> CheckAtPos/5
  Constant5/1 -> CheckAtPos/4
  Constant8/1 -> CheckAtPos3/5
  Constant7/1 -> CheckAtPos3/4
  Constant10/1 -> CheckAtPos4/5
  Constant9/1 -> CheckAtPos4/4
  [SecRwLtStBkReclnUpwdDnwdPosV] -> CheckAtPos2/2
  IsArrivedTarZone5/1 -> [Step1_6_ArrivedTarPos]
  [KeSMSuSecRwStHeadrestFwdBkwdPosDelta_Val] -> IsArrivedTarZone5/3
  [SecRwLtStHdrstFrwdBkwdPos] -> IsArrivedTarZone5/1
  [K_HdrstFrwdBkwdnwdPosMax] -> IsArrivedTarZone5/4
  [K_HdrstFrwdBkwdnwdPosMin] -> IsArrivedTarZone5/2
  Constant12/1 -> CheckAtPos5/4
  Constant11/1 -> CheckAtPos5/5
  [SecRwLtStHdrstFrwdBkwdPosV] -> CheckAtPos5/2
  [Step1_6_ArrivedTarPos] -> CheckAtPos5/3
  [HdrstFrwdBkwdMovConfig] -> CheckAtPos5/1
  CheckAtPos5/1 -> Logical Operator9/6  "LyL_Step1_6_ArrivedTarPos"
  Bus Selector5/4 -> [HdrstFrwdBkwdMovConfig]  "<HdrstFrwdBkwdMovConfig>"
  Bus Selector7/3 -> [SecRwLtStHdrstFrwdBkwdPosV]  "<IfVeSMSuSecRwLtStHdrstFrwdBkwdPosV_Val_read>"
  Bus Selector1/3 -> [SecRwLtStHdrstFrwdBkwdPos]  "<IfVeSMSuSecRwLtStHdrstFrwdBkwdPos_Val_read>"
  Multiport Switch/1 -> Bus Selector8/1, Calib_Ly4sLAdpt/1
  PA_KeSMSw4sLyingMDSecRwLtStHdrstFrwdBkwdnwdPosMin_165_Val/1 -> Bus Creator2/9  "HdrstFrwdBkwdnwdPosMin"
  PA_KeSMSw4sLyingMDSecRwLtStHdrstFrwdBkwdnwdPosMax_165_Val/1 -> Bus Creator2/8  "HdrstFrwdBkwdnwdPosMax"
  PA_KeSMSw4sLyingMDSecRwLtStHdrstFrwdBkwdnwdPos_165_Val/1 -> Bus Creator2/7  "HdrstFrwdBkwdnwdPos"
  PA_KeSMSw4sLyingMDSecRwLtStLgrstOtwdInwdPos_Below160_Val/1 -> Bus Creator/4  "LgrstOtwdInwdPos"
  PA_KeSMSw4sLyingMDSecRwLtStHdrstUpwdDnwdPosMax_160_Val/1 -> Bus Creator1/2  "HdrstUpwdDnwdPosMax"
  Bus Creator1/1 -> Multiport Switch/3  "Ly4sLAdpt"
  PA_KeSMSw4sLyingMDSecRwLtStHdrstUpwdDnwdPosMin_160_Val/1 -> Bus Creator1/3  "HdrstUpwdDnwdPosMin"
  PA_KeSMSw4sLyingMDSecRwLtStHdrstUpwdDnwdPosMin_165_Val/1 -> Bus Creator2/3  "HdrstUpwdDnwdPosMin"
  PA_KeSMSw4sLyingMDSecRwLtStHdrstUpwdDnwdPosMax_170_Val/1 -> Bus Creator3/2  "HdrstUpwdDnwdPosMax"
  PA_KeSMSw4sLyingMDSecRwLtStHdrstUpwdDnwdPos_165_Val/1 -> Bus Creator2/1  "HdrstUpwdDnwdPos"
  PA_KeSMSw4sLyingMDSecRwLtStLgrstOtwdInwdPos_165_Val/1 -> Bus Creator2/4  "LgrstOtwdInwdPos"
  PA_KeSMSw4sLyingMDSecRwLtStHdrstUpwdDnwdPos_170_Val/1 -> Bus Creator3/1  "HdrstUpwdDnwdPos"
  PA_KeSMSw4sLyingMDSecRwLtStLgrstOtwdInwdPosMin_180_Val/1 -> Bus Creator5/6  "LgrstOtwdInwdPosMin"
  PA_KeSMSw4sLyingMDSecRwLtStHdrstUpwdDnwdPos_180_Val/1 -> Bus Creator5/1  "HdrstUpwdDnwdPos"
  PA_KeSMSw4sLyingMDSecRwLtStLgrstOtwdInwdPosMax_160_Val/1 -> Bus Creator1/5  "LgrstOtwdInwdPosMax"
  PA_KeSMSw4sLyingMDSecRwLtStHdrstFrwdBkwdnwdPosMin_160_Val/1 -> Bus Creator1/9  "HdrstFrwdBkwdnwdPosMin"
  PA_KeSMSw4sLyingMDSecRwLtStHdrstFrwdBkwdnwdPos_160_Val/1 -> Bus Creator1/7  "HdrstFrwdBkwdnwdPos"
  PA_KeSMSw4sLyingMDSecRwLtStLgrstOtwdInwdPosMax_Below160_Val/1 -> Bus Creator/5  "LgrstOtwdInwdPosMax"
  PA_KeSMSw4sLyingMDSecRwLtStLgrstOtwdInwdPos_170_Val/1 -> Bus Creator3/4  "LgrstOtwdInwdPos"
  PA_KeSMSw4sLyingMDSecRwLtStHdrstFrwdBkwdnwdPosMax_160_Val/1 -> Bus Creator1/8  "HdrstFrwdBkwdnwdPosMax"
  PA_KeSMSw4sLyingMDSecRwLtStHdrstUpwdDnwdPosMin_180_Val/1 -> Bus Creator5/3  "HdrstUpwdDnwdPosMin"
  PA_KeSMSw4sLyingMDSecRwLtStLgrstOtwdInwdPosMin_170_Val/1 -> Bus Creator3/6  "LgrstOtwdInwdPosMin"
  PA_KeSMSw4sLyingMDSecRwLtStHdrstUpwdDnwdPosMax_175_Val/1 -> Bus Creator4/2  "HdrstUpwdDnwdPosMax"
  PA_KeSMSw4sLyingMDSecRwLtStHdrstUpwdDnwdPosMin_175_Val/1 -> Bus Creator4/3  "HdrstUpwdDnwdPosMin"
  PA_KeSMSw4sLyingMDSecRwLtStHdrstUpwdDnwdPos_175_Val/1 -> Bus Creator4/1  "HdrstUpwdDnwdPos"
  PA_KeSMSw4sLyingMDSecRwLtStLgrstOtwdInwdPosMin_160_Val/1 -> Bus Creator1/6  "LgrstOtwdInwdPosMin"
  PA_KeSMSw4sLyingMDSecRwLtStHdrstFrwdBkwdnwdPosMax_170_Val/1 -> Bus Creator3/8  "HdrstFrwdBkwdnwdPosMax"
  PA_KeSMSw4sLyingMDSecRwLtStHdrstFrwdBkwdnwdPosMin_170_Val/1 -> Bus Creator3/9  "HdrstFrwdBkwdnwdPosMin"
  Bus Creator/1 -> Multiport Switch/2  "Ly4sLAdpt"
  PA_KeSMSw4sLyingMDSecRwLtStHdrstFrwdBkwdnwdPosMin_Below160_Val/1 -> Bus Creator/9  "HdrstFrwdBkwdnwdPosMin"
  PA_KeSMSw4sLyingMDSecRwLtStLgrstOtwdInwdPosMax_175_Val/1 -> Bus Creator4/5  "LgrstOtwdInwdPosMax"
  PA_KeSMSw4sLyingMDSecRwLtStLgrstOtwdInwdPos_160_Val/1 -> Bus Creator1/4  "LgrstOtwdInwdPos"
  PA_KeSMSw4sLyingMDSecRwLtStHdrstFrwdBkwdnwdPos_Below160_Val/1 -> Bus Creator/7  "HdrstFrwdBkwdnwdPos"
  PA_KeSMSw4sLyingMDSecRwLtStHdrstUpwdDnwdPosMax_165_Val/1 -> Bus Creator2/2  "HdrstUpwdDnwdPosMax"
  PA_KeSMSw4sLyingMDSecRwLtStHdrstUpwdDnwdPosMin_Over180_Val/1 -> Bus Creator6/3  "HdrstUpwdDnwdPosMin"
  Bus Creator4/1 -> Multiport Switch/6  "Ly4sLAdpt"
  PA_KeSMSw4sLyingMDSecRwLtStHdrstUpwdDnwdPosMax_180_Val/1 -> Bus Creator5/2  "HdrstUpwdDnwdPosMax"
  PA_KeSMSw4sLyingMDSecRwLtStHdrstUpwdDnwdPosMax_Over180_Val/1 -> Bus Creator6/2  "HdrstUpwdDnwdPosMax"
  PA_KeSMSw4sLyingMDSecRwLtStHdrstFrwdBkwdnwdPos_170_Val/1 -> Bus Creator3/7  "HdrstFrwdBkwdnwdPos"
  PA_KeSMSw4sLyingMDSecRwLtStHdrstFrwdBkwdnwdPos_180_Val/1 -> Bus Creator5/7  "HdrstFrwdBkwdnwdPos"
  PA_KeSMSw4sLyingMDSecRwLtStHdrstFrwdBkwdnwdPosMin_180_Val/1 -> Bus Creator5/9  "HdrstFrwdBkwdnwdPosMin"
  PA_KeSMSw4sLyingMDSecRwLtStLgrstOtwdInwdPos_180_Val/1 -> Bus Creator5/4  "LgrstOtwdInwdPos"
  PA_KeSMSw4sLyingMDSecRwLtStHdrstFrwdBkwdnwdPosMax_180_Val/1 -> Bus Creator5/8  "HdrstFrwdBkwdnwdPosMax"
  PA_KeSMSw4sLyingMDSecRwLtStHdrstFrwdBkwdnwdPos_Over180_Val/1 -> Bus Creator6/7  "HdrstFrwdBkwdnwdPos"
  PA_KeSMSw4sLyingMDSecRwLtStHdrstFrwdBkwdnwdPosMin_Over180_Val/1 -> Bus Creator6/9  "HdrstFrwdBkwdnwdPosMin"
  PA_KeSMSw4sLyingMDSecRwLtStHdrstFrwdBkwdnwdPosMax_Over180_Val/1 -> Bus Creator6/8  "HdrstFrwdBkwdnwdPosMax"
  PA_KeSMSw4sLyingMDSecRwLtStHdrstFrwdBkwdnwdPosMax_Below160_Val/1 -> Bus Creator/8  "HdrstFrwdBkwdnwdPosMax"
  PA_KeSMSw4sLyingMDSecRwLtStLgrstOtwdInwdPos_175_Val/1 -> Bus Creator4/4  "LgrstOtwdInwdPos"
  Bus Creator2/1 -> Multiport Switch/4  "Ly4sLAdpt"
  PA_KeSMSw4sLyingMDSecRwLtStLgrstOtwdInwdPosMin_Over180_Val/1 -> Bus Creator6/6  "LgrstOtwdInwdPosMin"
  PA_KeSMSw4sLyingMDSecRwLtStHdrstUpwdDnwdPosMin_170_Val/1 -> Bus Creator3/3  "HdrstUpwdDnwdPosMin"
  PA_KeSMSw4sLyingMDSecRwLtStLgrstOtwdInwdPos_Over180_Val/1 -> Bus Creator6/4  "LgrstOtwdInwdPos"
  PA_KeSMSw4sLyingMDSecRwLtStHdrstUpwdDnwdPos_160_Val/1 -> Bus Creator1/1  "HdrstUpwdDnwdPos"
  PA_KeSMSw4sLyingMDSecRwLtStLgrstOtwdInwdPosMax_Over180_Val/1 -> Bus Creator6/5  "LgrstOtwdInwdPosMax"
  Bus Creator6/1 -> Multiport Switch/8  "Ly4sLAdpt"
  PA_KeSMSw4sLyingMDSecRwLtStLgrstOtwdInwdPosMax_180_Val/1 -> Bus Creator5/5  "LgrstOtwdInwdPosMax"
  PA_KeSMSw4sLyingMDSecRwLtStLgrstOtwdInwdPosMin_165_Val/1 -> Bus Creator2/6  "LgrstOtwdInwdPosMin"
  PA_KeSMSw4sLyingMDSecRwLtStLgrstOtwdInwdPosMax_170_Val/1 -> Bus Creator3/5  "LgrstOtwdInwdPosMax"
  PA_KeSMSw4sLyingMDSecRwLtStHdrstUpwdDnwdPos_Below160_Val/1 -> Bus Creator/1  "HdrstUpwdDnwdPos"
  PA_KeSMSw4sLyingMDSecRwLtStLgrstOtwdInwdPosMin_175_Val/1 -> Bus Creator4/6  "LgrstOtwdInwdPosMin"
  PA_KeSMSw4sLyingMDSecRwLtStHdrstFrwdBkwdnwdPosMin_175_Val/1 -> Bus Creator4/9  "HdrstFrwdBkwdnwdPosMin"
  Lt4sHightIndex/1 -> Multiport Switch/1
  Bus Creator3/1 -> Multiport Switch/5  "Ly4sLAdpt"
  PA_KeSMSw4sLyingMDSecRwLtStHdrstUpwdDnwdPosMin_Below160_Val/1 -> Bus Creator/3  "HdrstUpwdDnwdPosMin"
  PA_KeSMSw4sLyingMDSecRwLtStLgrstOtwdInwdPosMax_165_Val/1 -> Bus Creator2/5  "LgrstOtwdInwdPosMax"
  PA_KeSMSw4sLyingMDSecRwLtStHdrstFrwdBkwdnwdPos_175_Val/1 -> Bus Creator4/7  "HdrstFrwdBkwdnwdPos"
  PA_KeSMSw4sLyingMDSecRwLtStHdrstUpwdDnwdPos_Over180_Val/1 -> Bus Creator6/1  "HdrstUpwdDnwdPos"
  PA_KeSMSw4sLyingMDSecRwLtStHdrstFrwdBkwdnwdPosMax_175_Val/1 -> Bus Creator4/8  "HdrstFrwdBkwdnwdPosMax"
  Bus Creator5/1 -> Multiport Switch/7  "Ly4sLAdpt"
  PA_KeSMSw4sLyingMDSecRwLtStHdrstUpwdDnwdPosMax_Below160_Val/1 -> Bus Creator/2  "HdrstUpwdDnwdPosMax"
  PA_KeSMSw4sLyingMDSecRwLtStLgrstOtwdInwdPosMin_Below160_Val/1 -> Bus Creator/6  "LgrstOtwdInwdPosMin"
  Bus Selector8/1 -> [K_HdrstUpwdPosMax]  "<HdrstUpwdDnwdPosMax>"
  Bus Selector8/2 -> [K_HdrstUpwdPosMin]  "<HdrstUpwdDnwdPosMin>"
  Bus Selector8/3 -> [K_HdrstFrwdBkwdnwdPosMax]  "<HdrstFrwdBkwdnwdPosMax>"
  Bus Selector8/4 -> [K_HdrstFrwdBkwdnwdPosMin]  "<HdrstFrwdBkwdnwdPosMin>"
  Bus Selector8/5 -> [K_LgrstOtwdInwdPos_Max]  "<LgrstOtwdInwdPosMax>"
  Bus Selector8/6 -> [K_LgrstOtwdInwdPos_Min]  "<LgrstOtwdInwdPosMin>"
  Bus Selector2/3 -> [K_LgrstUpwdPosMax]  "<LgrstUpwdPosMax>"
  Bus Selector2/4 -> [K_LgrstUpwdPosMin]  "<LgrstUpwdPosMin>"
  Bus Selector9/5 -> [KeSMSuSecRwStBackPosDelta_Val]  "<KeSMSuSecRwStBackPosDelta_Val>"
  Bus Selector9/4 -> [KeSMSuSecRwStFtrstUpwdDnwdPosDelta_Val]  "<KeSMSuSecRwStFtrstUpwdDnwdPosDelta_Val>"
  Bus Selector9/6 -> [KeSMSuSecRwStLegrestUpwdDwnwdPosDelta_Val]  "<KeSMSuSecRwStLegrestUpwdDwnwdPosDelta_Val>"
  Bus Selector9/2 -> [KeSMSuSecRwStHeadrestUpwdDwnwdPosDelta_Val]  "<KeSMSuSecRwStHeadrestUpwdDwnwdPosDelta_Val>"
  Bus Selector9/3 -> [KeSMSuSecRwStLegrestInOutPosDelta_Val]  "<KeSMSuSecRwStLegrestInOutPosDelta_Val>"
  Bus Selector9/1 -> [KeSMSuSecRwStHeadrestFwdBkwdPosDelta_Val]  "<KeSMSuSecRwStHeadrestFwdBkwdPosDelta_Val>"
  PosDeltaCalib/1 -> Bus Selector9/1
